simulink model "Vehicle_Dynamic_Simulator"  (R2021b)
settings: Solver=VariableStepAuto  StartTime=0.0  StopTime=200  RelTol=1e-3
undefined symbols (not defined in the file): Path
libraries: Solver_SF x2, mpclib x1, sldrtlib x1
(part 2 of 2)

== matlab function Vehicle_Dynamic_Simulator/Estimation_Module/Whl_Fz_Estimation/Wheel_Kinematics_Estimation ==
  data: Delta_SW_Ref input; Whl_Kappa output; Veh_Vx_Ref input; Veh_Vy_Ref input; Veh_AVz_Ref input; Whl_Alpha output; Whl_AVy_Ref input
function [Whl_Kappa, Whl_Alpha] = ...
    Compute_Tyre_Kinematics(Delta_SW_Ref, Veh_Vx_Ref, Veh_Vy_Ref, Veh_AVz_Ref, Whl_AVy_Ref)
% Vehicle Parameters
     L  = [+1.265; +1.265; -1.895; -1.895];
     W  = [+0.802; -0.802; +0.802; -0.802];    
         
     R_whl = 0.368;
% Calculate Tyre Kinematic
    Whl_Vx = zeros(4,1);
    Whl_Vy = zeros(4,1);
     v_whl = zeros(4,1);

    Whl_Kappa = zeros(4,1);
    Whl_Alpha = zeros(4,1);

    for i = 1:1:4
        Whl_Vx(i,1) = + Veh_Vx_Ref - W(i,1)*Veh_AVz_Ref;
        Whl_Vy(i,1) = + Veh_Vy_Ref + L(i,1)*Veh_AVz_Ref;
         v_whl(i,1) = cos(Delta_SW_Ref(i,1))*sqrt(Whl_Vx(i,1)^2 + Whl_Vy(i,1)^2);

        Whl_Kappa(i,1) = (Whl_AVy_Ref(i,1)*R_whl - v_whl(i,1))/v_whl(i,1); 
        Whl_Alpha(i,1) = atan(Whl_Vy(i,1)/Whl_Vx(i,1)) - Delta_SW_Ref(i,1);
    end
end

== matlab function Vehicle_Dynamic_Simulator/Estimation_Module/Whl_Fx_Estimation/Wheel_Kinematics_Estimation ==
  data: Delta_SW_Ref input; Whl_Kappa output; Veh_Vx_Ref input; Veh_Vy_Ref input; Veh_AVz_Ref input; Whl_AVy_Ref input
function Whl_Kappa  = ...
    Compute_Tyre_Kinematics(Delta_SW_Ref, Veh_Vx_Ref, Veh_Vy_Ref, Veh_AVz_Ref, Whl_AVy_Ref)
% Vehicle Parameters
     L  = [+1.265; +1.265; -1.895; -1.895];
     W  = [+0.802; -0.802; +0.802; -0.802];    
         
     R_whl = 0.368;
% Calculate Tyre Kinematic
    Whl_Vx = zeros(4,1);
    Whl_Vy = zeros(4,1);
     v_whl = zeros(4,1);

    Whl_Kappa = zeros(4,1);
    Whl_Alpha = zeros(4,1);

    for i = 1:1:4
        Whl_Vx(i,1) = + Veh_Vx_Ref - W(i,1)*Veh_AVz_Ref;
        Whl_Vy(i,1) = + Veh_Vy_Ref + L(i,1)*Veh_AVz_Ref;
         v_whl(i,1) = cos(Delta_SW_Ref(i,1))*sqrt(Whl_Vx(i,1)^2 + Whl_Vy(i,1)^2);

        Whl_Kappa(i,1) = (Whl_AVy_Ref(i,1)*R_whl - v_whl(i,1))/v_whl(i,1); 
        Whl_Alpha(i,1) = atan(Whl_Vy(i,1)/Whl_Vx(i,1)) - Delta_SW_Ref(i,1);
    end
end

== matlab function Vehicle_Dynamic_Simulator/Estimation_Module/Whl_Fy_Estimation/Wheel_Kinematics_Estimation ==
  data: Delta_SW_Ref input; Whl_Kappa output; Veh_Vx_Ref input; Veh_Vy_Ref input; Veh_AVz_Ref input; Whl_AVy_Ref input
function Whl_Kappa  = ...
    Compute_Tyre_Kinematics(Delta_SW_Ref, Veh_Vx_Ref, Veh_Vy_Ref, Veh_AVz_Ref, Whl_AVy_Ref)
% Vehicle Parameters
     L  = [+1.265; +1.265; -1.895; -1.895];
     W  = [+0.802; -0.802; +0.802; -0.802];    
         
     R_whl = 0.368;
% Calculate Tyre Kinematic
    Whl_Vx = zeros(4,1);
    Whl_Vy = zeros(4,1);
     v_whl = zeros(4,1);

    Whl_Kappa = zeros(4,1);
    Whl_Alpha = zeros(4,1);

    for i = 1:1:4
        Whl_Vx(i,1) = + Veh_Vx_Ref - W(i,1)*Veh_AVz_Ref;
        Whl_Vy(i,1) = + Veh_Vy_Ref + L(i,1)*Veh_AVz_Ref;
         v_whl(i,1) = cos(Delta_SW_Ref(i,1))*sqrt(Whl_Vx(i,1)^2 + Whl_Vy(i,1)^2);

        Whl_Kappa(i,1) = (Whl_AVy_Ref(i,1)*R_whl - v_whl(i,1))/v_whl(i,1); 
        Whl_Alpha(i,1) = atan(Whl_Vy(i,1)/Whl_Vx(i,1)) - Delta_SW_Ref(i,1);
    end
end

== matlab function Vehicle_Dynamic_Simulator/Control_Module/Lat_Controller/Stanley_Controller/MATLAB Function2 ==
  data: K_feed output; Veh_Vx_Ref input
function K_feed  = Stanley_K_Interpolation(Veh_Vx_Ref)
    K_table = load("Controllers\Lateral_Controller\Stanley_Controller\Conf\Stanley_K_table.mat");
    K_table = K_table.Stanley_K_Table;
    K_feed  = interp1(K_table(:,2), K_table(:,3), Veh_Vx_Ref, 'linear', 'extrap');
end

== matlab function Vehicle_Dynamic_Simulator/Localization_Module/Error_Calculation/MATLAB Function ==
  data: Path_Theta_Est input; Path_Kappa_Est input; Path_L_Ref input; Veh_Yz_Ref input; Veh_Vx_Ref input; Veh_Vy_Ref input; Veh_AVz_Ref input; Veh_ErrY_Est output; Veh_ErrVy_Est output; Veh_ErrYz_Est output; Veh_ErrAVz_Est output
function [Veh_ErrY_Est, Veh_ErrVy_Est, Veh_ErrYz_Est, Veh_ErrAVz_Est] = ...
    Error_Calculate(Path_Theta_Est, ...
                    Path_Kappa_Est, ...
                    Path_L_Ref,     ...
                    Veh_Yz_Ref,     ...                  
                    Veh_Vx_Ref,     ...
                    Veh_Vy_Ref,     ...
                    Veh_AVz_Ref)
    Veh_ErrY_Est   = Path_L_Ref;
    Veh_ErrYz_Est  = Veh_Yz_Ref - Path_Theta_Est;
    Veh_ErrVy_Est  = Veh_Vy_Ref + Veh_Vx_Ref*Veh_ErrYz_Est;
    Veh_ErrAVz_Est = Veh_AVz_Ref - Veh_Vx_Ref*Path_Kappa_Est;
end

== matlab function Vehicle_Dynamic_Simulator/Localization_Module/Prev_Calculation/MATLAB Function1 ==
  data: Path_S_Ref input; ts input; Veh_Vx_Ref input; Path_S_Prev output
function Path_S_Prev = ComputePathSPrev(Path_S_Ref, ts,Veh_Vx_Ref)
    Path_S_Prev = zeros(201, 1);

    for i = 1:1:201
        Path_S_Prev(i, 1) = Path_S_Ref + (i-1)*ts*Veh_Vx_Ref;
    end
end

== matlab function Vehicle_Dynamic_Simulator/Control_Module/Lat_Controller/Offline_OPC_Controller/MATLAB Function2 ==
  data: K_feed output; Veh_Vx_Ref input; K_lag output; K_delay output; K_prev output
function [K_feed, K_lag, K_delay, K_prev] = OPC_K_Interpolation(Veh_Vx_Ref)
    K_table = load("Controllers\Lateral_Controller\Optimal_Preview_Controller\Conf\optimal_preview_K_table.mat");
    K_table = K_table.OPC_K_Table;
    
    K_total = zeros(1,226);

    for i=1:1:226
        K_total(1,i) = interp1(K_table(:,2), K_table(:,i+2), Veh_Vx_Ref, 'linear', 'extrap');
    end
    
    K_feed = K_total(1,1:4);
    K_lag  = K_total(1,5);
    K_delay= K_total(6:25);
    K_prev = K_total(26:226);
end

== matlab function Vehicle_Dynamic_Simulator/Estimation_Module/Whl_Alpha_Estimation/Wheel_Kinematics_Estimation ==
  data: Delta_SW_Ref input; Whl_Kappa output; Veh_Vx_Ref input; Veh_Vy_Ref input; Veh_AVz_Ref input; Whl_Alpha output; Whl_AVy_Ref input
function [Whl_Kappa, Whl_Alpha] = ...
    Compute_Tyre_Kinematics(Delta_SW_Ref, Veh_Vx_Ref, Veh_Vy_Ref, Veh_AVz_Ref, Whl_AVy_Ref)
% Vehicle Parameters
     L  = [+1.265; +1.265; -1.895; -1.895];
     W  = [+0.802; -0.802; +0.802; -0.802];    
         
     R_whl = 0.368;
% Calculate Tyre Kinematic
    Whl_Vx = zeros(4,1);
    Whl_Vy = zeros(4,1);
     v_whl = zeros(4,1);

    Whl_Kappa = zeros(4,1);
    Whl_Alpha = zeros(4,1);

    for i = 1:1:4
        Whl_Vx(i,1) = + Veh_Vx_Ref - W(i,1)*Veh_AVz_Ref;
        Whl_Vy(i,1) = + Veh_Vy_Ref + L(i,1)*Veh_AVz_Ref;
         v_whl(i,1) = cos(Delta_SW_Ref(i,1))*sqrt(Whl_Vx(i,1)^2 + Whl_Vy(i,1)^2);

        Whl_Kappa(i,1) = (Whl_AVy_Ref(i,1)*R_whl - v_whl(i,1))/v_whl(i,1); 
        Whl_Alpha(i,1) = atan(Whl_Vy(i,1)/Whl_Vx(i,1)) - Delta_SW_Ref(i,1);
    end
end

== matlab function Vehicle_Dynamic_Simulator/Estimation_Module/Whl_Kappa_Estimation/Wheel_Kinematics_Estimation ==
  data: Delta_SW_Ref input; Whl_Kappa output; Veh_Vx_Ref input; Veh_Vy_Ref input; Veh_AVz_Ref input; Whl_AVy_Ref input
function Whl_Kappa  = ...
    Compute_Tyre_Kinematics(Delta_SW_Ref, Veh_Vx_Ref, Veh_Vy_Ref, Veh_AVz_Ref, Whl_AVy_Ref)
% Vehicle Parameters
     L  = [+1.265; +1.265; -1.895; -1.895];
     W  = [+0.802; -0.802; +0.802; -0.802];    
         
     R_whl = 0.368;
% Calculate Tyre Kinematic
    Whl_Vx = zeros(4,1);
    Whl_Vy = zeros(4,1);
     v_whl = zeros(4,1);

    Whl_Kappa = zeros(4,1);
    Whl_Alpha = zeros(4,1);

    for i = 1:1:4
        Whl_Vx(i,1) = + Veh_Vx_Ref - W(i,1)*Veh_AVz_Ref;
        Whl_Vy(i,1) = + Veh_Vy_Ref + L(i,1)*Veh_AVz_Ref;
         v_whl(i,1) = cos(Delta_SW_Ref(i,1))*sqrt(Whl_Vx(i,1)^2 + Whl_Vy(i,1)^2);

        Whl_Kappa(i,1) = (Whl_AVy_Ref(i,1)*R_whl - v_whl(i,1))/v_whl(i,1); 
        Whl_Alpha(i,1) = atan(Whl_Vy(i,1)/Whl_Vx(i,1)) - Delta_SW_Ref(i,1);
    end
end

== matlab function Vehicle_Dynamic_Simulator/Estimation_Module/Vehicle_Model/7DOF_Model/MATLAB Function ==
  data: delta_whl input; kappa_whl output; vx_veh input; vy_veh input; avz_veh input; alpha_whl output; ax_veh output; ay_veh output; aaz_veh output; avy_whl input
function [kappa_whl, alpha_whl, ax_veh, ay_veh, aaz_veh] = ...
    Vehicle_Model(delta_whl, vx_veh, vy_veh, avz_veh, avy_whl)
% Vehicle Parameters
     W  = [+0.775; -0.775; +0.825; -0.825];    
     L  = [+0.970; +0.970; -1.810; -1.810];
     Kx = [+45000; +45000; +45000; +45000];      
     Ky = [-50000; -50000; -50000; -50000];    
     M  = 1521;                  
     Iz = 1816;          
     R_whl = 0.329;
% Calculate Tyre Kinematic
    vx_whl = zeros(4,1);
    vy_whl = zeros(4,1);
     v_whl = zeros(4,1);

    kappa_whl = zeros(4,1);
    alpha_whl = zeros(4,1);

    for i = 1:1:4
        vx_whl(i,1) = vx_veh - W(i,1)*avz_veh;
        vy_whl(i,1) = vy_veh + L(i,1)*avz_veh;
         v_whl(i,1) = cos(delta_whl(i,1))*sqrt(vx_whl(i,1)^2 + vy_whl(i,1)^2);

        kappa_whl(i,1) = (avy_whl(i,1)*R_whl - v_whl(i,1))/v_whl(i,1); 
        alpha_whl(i,1) = atan(vy_whl(i,1)/vx_whl(i,1)) - delta_whl(i,1);
    end

% Calculate State   
     ax_veh =  vy_veh*avz_veh;
     ay_veh = -vx_veh*avz_veh;
    aaz_veh = 0;
    for j = 1:1:4
        ax_veh = ax_veh + ...
            (1/M)*(Kx(i,1)*kappa_whl(i,1)*cos(delta_whl(i,1)) - ...
                   Ky(i,1)*alpha_whl(i,1)*sin(delta_whl(i,1)));
        ay_veh = ay_veh + ...
            (1/M)*(Kx(i,1)*kappa_whl(i,1)*sin(delta_whl(i,1)) + ...
                   Ky(i,1)*alpha_whl(i,1)*cos(delta_whl(i,1)));
        aaz_veh = aaz_veh + ...
            (1/Iz)*(-W(i,1))*...
            (Kx(i,1)*kappa_whl(i,1)*cos(delta_whl(i,1)) - ...
             Ky(i,1)*alpha_whl(i,1)*sin(delta_whl(i,1))) + ...
            (1/Iz)*(L(i,1))*...
            (Kx(i,1)*kappa_whl(i,1)*sin(delta_whl(i,1)) - ...
             Ky(i,1)*alpha_whl(i,1)*cos(delta_whl(i,1)));
    end
end
